simulink subsystem "long_deg_to_km"  (R2022a)
settings: Solver=VariableStepAuto  StartTime=0.0  StopTime=10.0  RelTol=1e-3
settings Model: Creator=rodri  LastModifiedBy=rodri

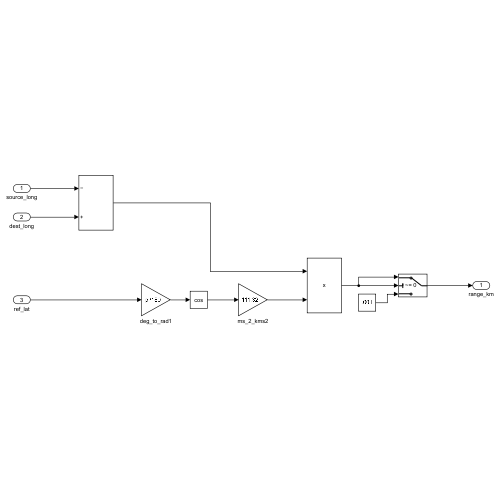
[thumbnail: Simulink's stored preview of the top-level diagram]
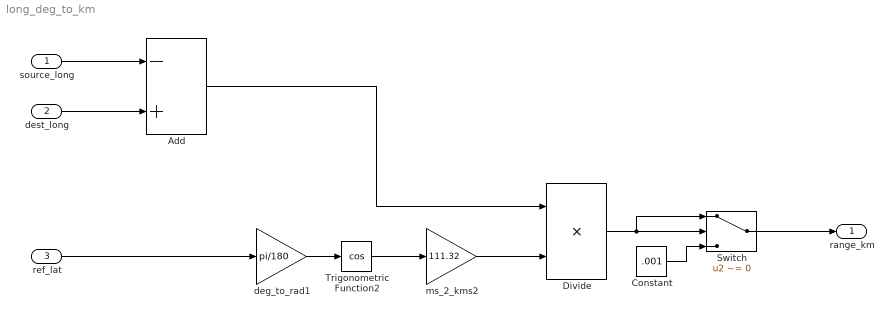
== system long_deg_to_km ==
  source_long : Inport
  dest_long : Inport  Port=2
  ref_lat : Inport  Port=3
  Add : Sum  Inputs=-+
  Constant : Constant  Value=.001
  Divide : Product  Inputs=**
  Switch : Switch  Criteria=u2 ~= 0  SaturateOnIntegerOverflow=off  InputSameDT=off
  Trigonometric Function2 : Trigonometry  Operator=cos
  deg_to_rad1 : Gain  Gain=pi/180
  ms_2_kms2 : Gain  Gain=111.32
  range_km : Outport
  wires:
  deg_to_rad1/1 -> Trigonometric Function2/1
  ref_lat/1 -> deg_to_rad1/1
  Divide/1 -> Switch/1, Switch/2
  ms_2_kms2/1 -> Divide/2
  Trigonometric Function2/1 -> ms_2_kms2/1
  source_long/1 -> Add/1
  Constant/1 -> Switch/3
  Switch/1 -> range_km/1
  Add/1 -> Divide/1
  dest_long/1 -> Add/2
